simulink model "BMS_M0_pack_pass2"  (R2026a)
settings: Solver=VariableStepAuto  AbsTol=1e-3  EnableMultiTasking=on
undefined symbols (not defined in the file or in its folder): bat, mcu
libraries: fl_lib x22, nesl_utility x18, batteryecm_lib x6, ee_lib x4
settings SimscapeCC: SimscapeNominalValues="[{\"value\":\"1\",\"unit\":\"A\"},{\"value\":\"1\",\"unit\":\"bar\"},{\"value\":\"1\",\"unit\":\"cm^2\"},{\"value\":\"1\",\"unit\":\"cm^3/s\"},{\"value\":\"1\",\"unit\":\"kJ/kg\"},{\"value\":\"1\",\"unit\":\"kW\"},{\"value\":\"1\",\"unit\":\"l\"},{\"value\":\"1\",\"unit\":\"N\"},{\"value\":\"1\",\"unit\":\"N*m\"},{\"value\":\"1\",\"unit\":\"V\"}]"

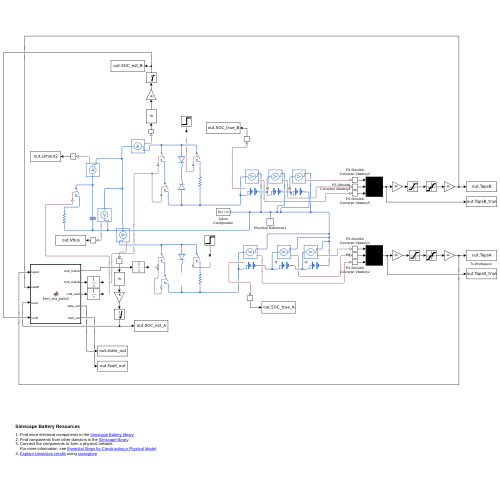
[thumbnail: Simulink's stored preview of the top-level diagram]
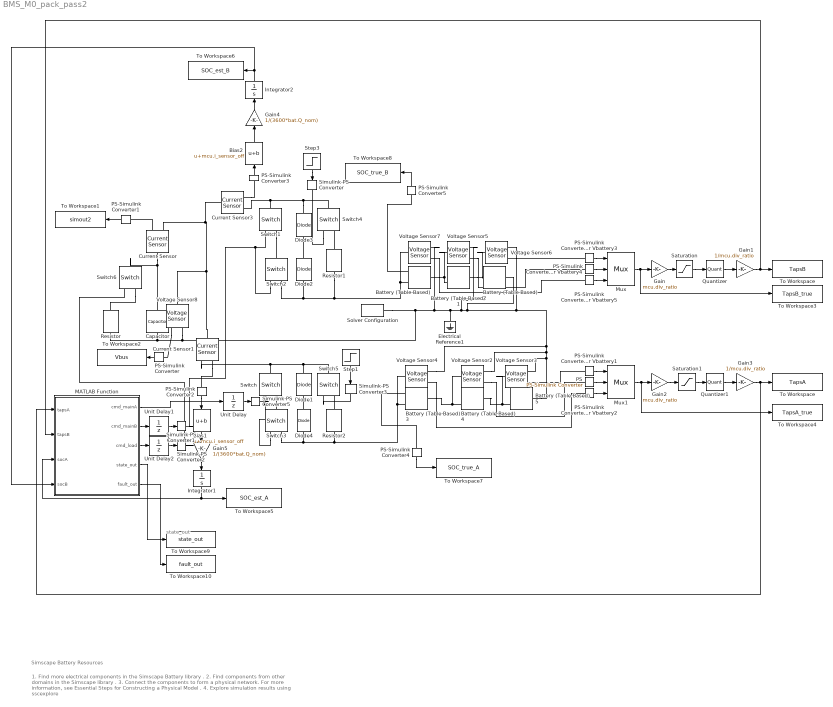
== system BMS_M0_pack_pass2 ==
  note: 1. Find more electrical components in the Simscape Battery library .
      | 2. Find components from other domains in the Simscape library .
      | 3. Connect the components to form a physical network.
      | For more information, see Essential Steps for Constructing a Physical Model .
      | 4. Explore simulation results using sscexplore
  note: Simscape Battery Resources
  note: state_out
  Battery (Table-Based){,1..3,5} (5 alike) : batteryecm_lib/Battery (Table-Based)  SOC_vec=bat.SOC_bp  T_dependence=simscape.enum.tablebattery.temperature_dependence.no  prm_dir=simscape.enum.tablebattery.prm_dir.noCurrentDirectionality  T_vec=[278, 293, 313] K  V0_mat=[3.49, 3.5, 3.51; 3.55, 3.57, 3.56; 3.62, 3.63, 3.64; 3.71, 3.71, 3.72; 3.91, 3.93, 3.94; 4.07, 4.08, 4.08; 4.19, 4.19, 4.19] V  V0_vec=bat.OCV_tbl V  V_range=[0, inf] V  R0_mat=[.0117, .0085, .009; .011, .0085, .009; .0114, .0087, .0092; .0107, .0082, .0088; .0107, .0083, .0091; .0113, .0085, .0089; .0116, .0085, .0089] Ohm  R0_vec=bat.R0 * ones(size(bat.SOC_bp)) Ohm  R0_dis_mat=[.0117, .0085, .009; .011, .0085, .009; .0114, .0087, .0092; .0107, .0082, .0088; .0107, .0083, .0091; .0113, .0085, .0089; .0116, .0085, .0089] Ohm  R0_dis_vec=[.0085, .0085, .0087, .0082, .0083, .0085, .0085] Ohm  R0_ch_mat=[.0117, .0085, .009; .011, .0085, .009; .0114, .0087, .0092; .0107, .0082, .0088; .0107, .0083, .0091; .0113, .0085, .0089; .0116, .0085, .0089] Ohm  R0_ch_vec=[.0085, .0085, .0087, .0082, .0083, .0085, .0085] Ohm  AH=bat.Q_nom A*hr  prm_leak=simscape.enum.tablebattery.prm_leak.disabled  Rleak_vec=[8000, 7000, 6000] Ohm  Rleak=7e3 Ohm  extrapolation_option=simscape.enum.extrapolation.nearest  SOC_port=simscape.enum.tablebattery.enable.yes  prm_dyn=simscape.enum.tablebattery.prm_dyn.off  R1_mat=[.0109, .0029, .0013; .0069, .0024, .0012; .0047, .0026, .0013; .0034, .0016, .001; .0033, .0023, .0014; .0033, .0018, .0011; .0028, .0017, .0011] Ohm  R1_vec=[.0029, .0024, .0026, .0016, .0023, .0018, .0017] Ohm  tau1_mat=[20, 36, 39; 31, 45, 39; 109, 105, 61; 36, 29, 26; 59, 77, 67; 40, 33, 29; 25, 39, 33] s  tau1_vec=[36, 45, 105, 29, 77, 33, 39] s  R2_mat=[.0109, .0029, .0013; .0069, .0024, .0012; .0047, .0026, .0013; .0034, .0016, .001; .0033, .0023, .0014; .0033, .0018, .0011; .0028, .0017, .0011] Ohm  R2_vec=[.0029, .0024, .0026, .0016, .0023, .0018, .0017] Ohm  tau2_mat=[20, 36, 39; 31, 45, 39; 109, 105, 61; 36, 29, 26; 59, 77, 67; 40, 33, 29; 25, 39, 33] s  tau2_vec=[36, 45, 105, 29, 77, 33, 39] s  R3_mat=[.0109, .0029, .0013; .0069, .0024, .0012; .0047, .0026, .0013; .0034, .0016, .001; .0033, .0023, .0014; .0033, .0018, .0011; .0028, .0017, .0011] Ohm  R3_vec=[.0029, .0024, .0026, .0016, .0023, .0018, .0017] Ohm  tau3_mat=[20, 36, 39; 31, 45, 39; 109, 105, 61; 36, 29, 26; 59, 77, 67; 40, 33, 29; 25, 39, 33] s  tau3_vec=[36, 45, 105, 29, 77, 33, 39] s  R4_mat=[.0109, .0029, .0013; .0069, .0024, .0012; .0047, .0026, .0013; .0034, .0016, .001; .0033, .0023, .0014; .0033, .0018, .0011; .0028, .0017, .0011] Ohm  R4_vec=[.0029, .0024, .0026, .0016, .0023, .0018, .0017] Ohm  tau4_mat=[20, 36, 39; 31, 45, 39; 109, 105, 61; 36, 29, 26; 59, 77, 67; 40, 33, 29; 25, 39, 33] s  tau4_vec=[36, 45, 105, 29, 77, 33, 39] s  R5_mat=[.0109, .0029, .0013; .0069, .0024, .0012; .0047, .0026, .0013; .0034, .0016, .001; .0033, .0023, .0014; .0033, .0018, .0011; .0028, .0017, .0011] Ohm  R5_vec=[.0029, .0024, .0026, .0016, .0023, .0018, .0017] Ohm  tau5_mat=[20, 36, 39; 31, 45, 39; 109, 105, 61; 36, 29, 26; 59, 77, 67; 40, 33, 29; 25, 39, 33] s  tau5_vec=[36, 45, 105, 29, 77, 33, 39] s  prm_fade=simscape.enum.tablebattery.prm_fade.disabled  N0=100  dV0=0  dR0=0  dAH=0  dRleak=0  dR1=0  dR2=0  dR3=0  dR4=0  dR5=0  N0vec=[0, 100, 200, 300]  Tfadevec=[298.15, 323.15] K  dV0vec=[0, 0, 0, 0]  dR0vec=[0, 0, 0, 0]  dAHvec=[0, 0, 0, 0]  dRleakvec=[0, 0, 0, 0]  dR1vec=[0, 0, 0, 0]  dR2vec=[0, 0, 0, 0]  dR3vec=[0, 0, 0, 0]  dR4vec=[0, 0, 0, 0]  dR5vec=[0, 0, 0, 0]  dV0mat=[0, 0; 0, 0; 0, 0; 0, 0]  dR0mat=[0, 0; 0, 0; 0, 0; 0, 0]  dAHmat=[0, 0; 0, 0; 0, 0; 0, 0]  dRleakmat=[0, 0; 0, 0; 0, 0; 0, 0]  dR1mat=[0, 0; 0, 0; 0, 0; 0, 0]  dR2mat=[0, 0; 0, 0; 0, 0; 0, 0]  dR3mat=[0, 0; 0, 0; 0, 0; 0, 0]  dR4mat=[0, 0; 0, 0; 0, 0; 0, 0]  dR5mat=[0, 0; 0, 0; 0, 0; 0, 0]  prm_age_modeling=simscape.enum.tablebattery.prm_age_modeling.equation  storage_dt_age_vec=[0] d  storage_T_age_vec=[273] K  prm_age_OCV=simscape.enum.tablebattery.prm_age_OCV.OCV  OCV_age=0.9  SOC_age=0.6  prm_age_resistance=simscape.enum.tablebattery.prm_age.disabled  OCV_scaling_age_resistance=2.2134e6  OCV_offset_age_resistance=1.632e6  temp_exp_age_resistance=0.515833569 V  t_exp_age_resistance=0.75  T_age_vec_resistance=[273.15, 298.15, 323.15] K  dt_age_vec_resistance=[0, 90, 180, 270] d  dR0_age_vec=[0, 0, 0]  t_meas_dR0_age=100 d  dR0_age_mat=[0, 0, 0; 0, 0, 0; 0, 0, 0; 0, 0, 0]  prm_age_capacity=simscape.enum.tablebattery.prm_age.disabled  OCV_scaling_age_capacity=1.5097e07  OCV_offset_age_capacity=8.3625e06  temp_exp_age_capacity=0.6011 V  t_exp_age_capacity=0.75  T_age_vec_capacity=[273.15, 298.15, 323.15] K  dt_age_vec_capacity=[0, 90, 180, 270] d  dAH_age_vec=[0, 0, 0]  t_meas_dAH_age=100 d  dAH_age_mat=[0, 0, 0; 0, 0, 0; 0, 0, 0; 0, 0, 0]  thermal_port=simscape.enum.thermaleffects.omit  temperature=298.15 K  thermal_mass=100 J/K  i_specify=off  i_priority=None  i=0 A  i_nominal_specify=off  i_nominal_value=1  i_nominal_unit=A  v_specify=off  v_priority=None  v=0 V  v_nominal_specify=off  v_nominal_value=1  v_nominal_unit=V  stateOfCharge_specify=on  stateOfCharge_priority=High  stateOfCharge=0.50  stateOfCharge_nominal_specify=off  stateOfCharge_nominal_value=1  stateOfCharge_nominal_unit=1  num_cycles_specify=off  num_cycles_priority=High  num_cycles=0  num_cycles_nominal_specify=off  num_cycles_nominal_value=1  num_cycles_nominal_unit=1  cell_temperature_specify=off  cell_temperature_priority=High  cell_temperature=298.15 K  cell_temperature_nominal_specify=off  cell_temperature_nominal_value=1  cell_temperature_nominal_unit=K
      settings: LibrarySourceBlock=|
      | batt_lib/Cells/Battery
      | (Table-Based)
  Battery (Table-Based)4 : batteryecm_lib/Battery (Table-Based)  SOC_vec=bat.SOC_bp  T_dependence=simscape.enum.tablebattery.temperature_dependence.no  prm_dir=simscape.enum.tablebattery.prm_dir.noCurrentDirectionality  T_vec=[278, 293, 313] K  V0_mat=[3.49, 3.5, 3.51; 3.55, 3.57, 3.56; 3.62, 3.63, 3.64; 3.71, 3.71, 3.72; 3.91, 3.93, 3.94; 4.07, 4.08, 4.08; 4.19, 4.19, 4.19] V  V0_vec=bat.OCV_tbl V  V_range=[0, inf] V  R0_mat=[.0117, .0085, .009; .011, .0085, .009; .0114, .0087, .0092; .0107, .0082, .0088; .0107, .0083, .0091; .0113, .0085, .0089; .0116, .0085, .0089] Ohm  R0_vec=bat.R0 * ones(size(bat.SOC_bp)) Ohm  R0_dis_mat=[.0117, .0085, .009; .011, .0085, .009; .0114, .0087, .0092; .0107, .0082, .0088; .0107, .0083, .0091; .0113, .0085, .0089; .0116, .0085, .0089] Ohm  R0_dis_vec=[.0085, .0085, .0087, .0082, .0083, .0085, .0085] Ohm  R0_ch_mat=[.0117, .0085, .009; .011, .0085, .009; .0114, .0087, .0092; .0107, .0082, .0088; .0107, .0083, .0091; .0113, .0085, .0089; .0116, .0085, .0089] Ohm  R0_ch_vec=[.0085, .0085, .0087, .0082, .0083, .0085, .0085] Ohm  AH=bat.Q_nom A*hr  prm_leak=simscape.enum.tablebattery.prm_leak.disabled  Rleak_vec=[8000, 7000, 6000] Ohm  Rleak=7e3 Ohm  extrapolation_option=simscape.enum.extrapolation.nearest  SOC_port=simscape.enum.tablebattery.enable.yes  prm_dyn=simscape.enum.tablebattery.prm_dyn.off  R1_mat=[.0109, .0029, .0013; .0069, .0024, .0012; .0047, .0026, .0013; .0034, .0016, .001; .0033, .0023, .0014; .0033, .0018, .0011; .0028, .0017, .0011] Ohm  R1_vec=[.0029, .0024, .0026, .0016, .0023, .0018, .0017] Ohm  tau1_mat=[20, 36, 39; 31, 45, 39; 109, 105, 61; 36, 29, 26; 59, 77, 67; 40, 33, 29; 25, 39, 33] s  tau1_vec=[36, 45, 105, 29, 77, 33, 39] s  R2_mat=[.0109, .0029, .0013; .0069, .0024, .0012; .0047, .0026, .0013; .0034, .0016, .001; .0033, .0023, .0014; .0033, .0018, .0011; .0028, .0017, .0011] Ohm  R2_vec=[.0029, .0024, .0026, .0016, .0023, .0018, .0017] Ohm  tau2_mat=[20, 36, 39; 31, 45, 39; 109, 105, 61; 36, 29, 26; 59, 77, 67; 40, 33, 29; 25, 39, 33] s  tau2_vec=[36, 45, 105, 29, 77, 33, 39] s  R3_mat=[.0109, .0029, .0013; .0069, .0024, .0012; .0047, .0026, .0013; .0034, .0016, .001; .0033, .0023, .0014; .0033, .0018, .0011; .0028, .0017, .0011] Ohm  R3_vec=[.0029, .0024, .0026, .0016, .0023, .0018, .0017] Ohm  tau3_mat=[20, 36, 39; 31, 45, 39; 109, 105, 61; 36, 29, 26; 59, 77, 67; 40, 33, 29; 25, 39, 33] s  tau3_vec=[36, 45, 105, 29, 77, 33, 39] s  R4_mat=[.0109, .0029, .0013; .0069, .0024, .0012; .0047, .0026, .0013; .0034, .0016, .001; .0033, .0023, .0014; .0033, .0018, .0011; .0028, .0017, .0011] Ohm  R4_vec=[.0029, .0024, .0026, .0016, .0023, .0018, .0017] Ohm  tau4_mat=[20, 36, 39; 31, 45, 39; 109, 105, 61; 36, 29, 26; 59, 77, 67; 40, 33, 29; 25, 39, 33] s  tau4_vec=[36, 45, 105, 29, 77, 33, 39] s  R5_mat=[.0109, .0029, .0013; .0069, .0024, .0012; .0047, .0026, .0013; .0034, .0016, .001; .0033, .0023, .0014; .0033, .0018, .0011; .0028, .0017, .0011] Ohm  R5_vec=[.0029, .0024, .0026, .0016, .0023, .0018, .0017] Ohm  tau5_mat=[20, 36, 39; 31, 45, 39; 109, 105, 61; 36, 29, 26; 59, 77, 67; 40, 33, 29; 25, 39, 33] s  tau5_vec=[36, 45, 105, 29, 77, 33, 39] s  prm_fade=simscape.enum.tablebattery.prm_fade.disabled  N0=100  dV0=0  dR0=0  dAH=0  dRleak=0  dR1=0  dR2=0  dR3=0  dR4=0  dR5=0  N0vec=[0, 100, 200, 300]  Tfadevec=[298.15, 323.15] K  dV0vec=[0, 0, 0, 0]  dR0vec=[0, 0, 0, 0]  dAHvec=[0, 0, 0, 0]  dRleakvec=[0, 0, 0, 0]  dR1vec=[0, 0, 0, 0]  dR2vec=[0, 0, 0, 0]  dR3vec=[0, 0, 0, 0]  dR4vec=[0, 0, 0, 0]  dR5vec=[0, 0, 0, 0]  dV0mat=[0, 0; 0, 0; 0, 0; 0, 0]  dR0mat=[0, 0; 0, 0; 0, 0; 0, 0]  dAHmat=[0, 0; 0, 0; 0, 0; 0, 0]  dRleakmat=[0, 0; 0, 0; 0, 0; 0, 0]  dR1mat=[0, 0; 0, 0; 0, 0; 0, 0]  dR2mat=[0, 0; 0, 0; 0, 0; 0, 0]  dR3mat=[0, 0; 0, 0; 0, 0; 0, 0]  dR4mat=[0, 0; 0, 0; 0, 0; 0, 0]  dR5mat=[0, 0; 0, 0; 0, 0; 0, 0]  prm_age_modeling=simscape.enum.tablebattery.prm_age_modeling.equation  storage_dt_age_vec=[0] d  storage_T_age_vec=[273] K  prm_age_OCV=simscape.enum.tablebattery.prm_age_OCV.OCV  OCV_age=0.9  SOC_age=0.6  prm_age_resistance=simscape.enum.tablebattery.prm_age.disabled  OCV_scaling_age_resistance=2.2134e6  OCV_offset_age_resistance=1.632e6  temp_exp_age_resistance=0.515833569 V  t_exp_age_resistance=0.75  T_age_vec_resistance=[273.15, 298.15, 323.15] K  dt_age_vec_resistance=[0, 90, 180, 270] d  dR0_age_vec=[0, 0, 0]  t_meas_dR0_age=100 d  dR0_age_mat=[0, 0, 0; 0, 0, 0; 0, 0, 0; 0, 0, 0]  prm_age_capacity=simscape.enum.tablebattery.prm_age.disabled  OCV_scaling_age_capacity=1.5097e07  OCV_offset_age_capacity=8.3625e06  temp_exp_age_capacity=0.6011 V  t_exp_age_capacity=0.75  T_age_vec_capacity=[273.15, 298.15, 323.15] K  dt_age_vec_capacity=[0, 90, 180, 270] d  dAH_age_vec=[0, 0, 0]  t_meas_dAH_age=100 d  dAH_age_mat=[0, 0, 0; 0, 0, 0; 0, 0, 0; 0, 0, 0]  thermal_port=simscape.enum.thermaleffects.omit  temperature=298.15 K  thermal_mass=100 J/K  i_specify=off  i_priority=None  i=0 A  i_nominal_specify=off  i_nominal_value=1  i_nominal_unit=A  v_specify=off  v_priority=None  v=0 V  v_nominal_specify=off  v_nominal_value=1  v_nominal_unit=V  stateOfCharge_specify=on  stateOfCharge_priority=High  stateOfCharge=0.20  stateOfCharge_nominal_specify=off  stateOfCharge_nominal_value=1  stateOfCharge_nominal_unit=1  num_cycles_specify=off  num_cycles_priority=High  num_cycles=0  num_cycles_nominal_specify=off  num_cycles_nominal_value=1  num_cycles_nominal_unit=1  cell_temperature_specify=off  cell_temperature_priority=High  cell_temperature=298.15 K  cell_temperature_nominal_specify=off  cell_temperature_nominal_value=1  cell_temperature_nominal_unit=K
      settings: LibrarySourceBlock=|
      | batt_lib/Cells/Battery
      | (Table-Based)
  Bias1 : Bias  Bias=mcu.i_sensor_off  SaturateOnIntegerOverflow=off
  Bias2 : Bias  Bias=mcu.i_sensor_off  SaturateOnIntegerOverflow=off
  Capacitor : fl_lib/Electrical/Electrical Elements/Capacitor  c=1000 uF  r=1e-6 Ohm  g=0 1/Ohm  i_specify=off  i_priority=None  i=0 A  i_nominal_specify=off  i_nominal_value=1  i_nominal_unit=A  v_specify=off  v_priority=None  v=0 V  v_nominal_specify=off  v_nominal_value=1  v_nominal_unit=V  vc_specify=off  vc_priority=High  vc=0 V  vc_nominal_specify=off  vc_nominal_value=1  vc_nominal_unit=V
  Current Sensor : fl_lib/Electrical/Electrical Sensors/Current Sensor
  Current Sensor1 : fl_lib/Electrical/Electrical Sensors/Current Sensor
  Current Sensor3 : fl_lib/Electrical/Electrical Sensors/Current Sensor
  Diode{1..4} (4 alike) : ee_lib/Semiconductors & Converters/Diode  ModelType=ee.enum.diode.modelType.pwl  TableType=ee.enum.diode.tableType.IfMat  IfMat=[.07, .12, .19, 1.75, 4.24, 7.32, 11.2; .16, .3, .72, 2.14, 5.02, 8.35, 13.12] A  VfMat=[.9, 1.15, 1.25, 1.5, 1.75, 2.17, 2.6, 2.85; .58, .68, .75, 1.1, 1.38, 1.77, 2.27, 2.7] V  TjVec=[25, 125] degC  VfVec=[.5, .7, .9, 1.3, 1.7, 2.1, 2.5] V  IfVec=[.1, .2, .5, 1, 2, 4, 7, 10] A  IrMat=[1e-06, 2e-06, 5e-06, 1e-05, 2.5e-05, 5e-05, .0001; 2e-06, 5e-06, 1e-05, 4e-05, 8e-05, .0002, .0005] A  VrMat=[10, 100, 200, 250, 300, 325, 350; 10, 70, 160, 220, 270, 300, 320] V  VrVec=[10, 20, 40, 50, 70, 80, 100] V  IrVec=[1e-06, 2e-06, 5e-06, 1e-05, 2e-05, 5e-05, .0001] A  Vf=0.8 V  Ron=0.01 Ohm  Goff=1e-8 S  prmExp=ee.enum.diode.expParam.useTwo  I12=[.0137, .545] A  V12=[.6, .7] V  RS=0 Ohm  Tmeas=298.15 K  IS=1e-12 A  ec=1  I1=0.0137 A  V1=0.6 V  N_series=1  N_parallel=1  ZenerEnable=false  Rz=0.3 Ohm  BV=30 V  C_param=ee.enum.diode.capParam.fixed  CJ=0 pF  CJ0=5 pF  Vvec=[.1, 10, 100] V  Cvec=[3.5, 1, .4] pF  VJ=1 V  Mgrad=0.5  FC=0.5  Q_param=ee.enum.diode.recoveryParam.off  iRM=-7.15 A  iF=4 A  didt=-750 A/us  trr_factor=3  trr=115 ns  Qrr=150 nA*s  Vr=-600 V  Ls=150 nH  Erec=0.03 J  TT=50 ns  tau=100 ns  T_param=ee.enum.diode.temperatureParam.off  Tdevice=298.15 K  I1_T2=0.245 A  V1_T2=0.5 V  IS_T2=1.25e-7 A  Tmeas2=125 degC  XTI_param=ee.enum.diode.xtiParam.pn  XTI=3  EG_param=ee.enum.diode.egapParam.material_si  EG=1.11 eV  dBVdT=0 V/K  enable_fault_input=simscape.enum.onoff.off  i_specify=off  i_priority=None  i=0 A  i_nominal_specify=off  i_nominal_value=1  i_nominal_unit=A  v_specify=off  v_priority=None  v=0 V  v_nominal_specify=off  v_nominal_value=1  v_nominal_unit=V  v_capacitor_specify=off  v_capacitor_priority=None  v_capacitor=0 V  v_capacitor_nominal_specify=off  v_capacitor_nominal_value=1  v_capacitor_nominal_unit=V  Qj_specify=off  Qj_priority=High  Qj=0 C  Qj_nominal_specify=off  Qj_nominal_value=1  Qj_nominal_unit=C  i_diode_specify=off  i_diode_priority=None  i_diode=0 A  i_diode_nominal_specify=off  i_diode_nominal_value=1  i_diode_nominal_unit=A  v_diode_specify=off  v_diode_priority=None  v_diode=0 V  v_diode_nominal_specify=off  v_diode_nominal_value=1  v_diode_nominal_unit=V  i_capacitor_specify=off  i_capacitor_priority=None  i_capacitor=0 A  i_capacitor_nominal_specify=off  i_capacitor_nominal_value=1  i_capacitor_nominal_unit=A  fidelity_level=ee.enum.diode.fidelity.includeChargeDyn  rec_loss_model=ee.enum.diode.reverseRecoveryModelTabulateUpTo3D.fixed  ErecVal=0 J  scaleWithIandV=true  ErecMat=zeros(2, 3) J  ErecMat3D=zeros(2, 3, 2) J  TjrecVec=[298.15, 398.15] K  IfrecVec=[.1, 1, 10] A  IrecVal=10 A  VrecVal=10 V  VrecVec=[0, 100] V  tFilter=1 / 1000 / 100 s  thermal_network_parameterization=ee.enum.thermalNetworkTopology.junctionCase  Rth=[0, 10] K/W  Rth_Cauer=[1, 3, 10] K/W  Rth_Foster=[.08, .14, .22, .16] K/W  thermal_mass_parameterization=ee.enum.thermalNetwork.timeconstant  thermal_mass=[0, 1] J/K  thermal_mass_Cauer=[.1, .3, 1] J/K  thermal_mass_Foster=[.001, .005, .05, .5] J/K  thermal_time_constant=[0, 10] s  thermal_time_constant_Cauer=[1, 3, 10] s  thermal_time_constant_Foster=[7e-05, .0007, .01, .08] s  thermal_mass_initial_temperatures=[25, 25] degC  thermal_mass_initial_temperatures_Cauer=[25, 25, 25] degC  junction_thermal_mass=0.01 J/K  Tvec_initial_Foster=[25, 25, 25, 25] degC  no_thermal_network=0  junction_temperature_specify=off  junction_temperature_priority=None  junction_temperature=25 degC  junction_temperature_nominal_specify=off  junction_temperature_nominal_value=1  junction_temperature_nominal_unit=degC
  Electrical Reference1 : fl_lib/Electrical/Electrical Elements/Electrical Reference
  Gain : Gain  Gain=mcu.div_ratio
  Gain1 : Gain  Gain=1/mcu.div_ratio
  Gain2 : Gain  Gain=mcu.div_ratio
  Gain3 : Gain  Gain=1/mcu.div_ratio
  Gain4 : Gain  Gain=1/(3600*bat.Q_nom)
  Gain5 : Gain  Gain=1/(3600*bat.Q_nom)
  Integrator1 : Integrator  InitialCondition=0.55  LimitOutput=on  UpperSaturationLimit=1  LowerSaturationLimit=0
  Integrator2 : Integrator  InitialCondition=0.55  LimitOutput=on  UpperSaturationLimit=1  LowerSaturationLimit=0
  MATLAB Function : MATLAB Function  TreatAsAtomicUnit=on  SystemSampleTime=0.1
  Mux : Mux  Inputs=3
  Mux1 : Mux  Inputs=3
  PS : nesl_utility/PS-Simulink Converter  PhysicalDomain=network_engine_domain  SubClassName=ps_output  LeftPortType=input  RightPortType=output  PseudoPeriodic=off  Frequencies=[]  VectorFormat=inherit  Unit=inherit  AffineConversion=off
  PS-Simulink Converter{,1..5} (6 alike) : nesl_utility/PS-Simulink Converter  PhysicalDomain=network_engine_domain  SubClassName=ps_output  LeftPortType=input  RightPortType=output  PseudoPeriodic=off  Frequencies=[]  VectorFormat=inherit  Unit=inherit  AffineConversion=off
  PS-Simulink Converter Vbattery{1..5} (5 alike) : nesl_utility/PS-Simulink Converter  PhysicalDomain=network_engine_domain  SubClassName=ps_output  LeftPortType=input  RightPortType=output  PseudoPeriodic=off  Frequencies=[]  VectorFormat=inherit  Unit=inherit  AffineConversion=off
  Quantizer : Quantizer  QuantizationInterval=mcu.lsb_adc
  Quantizer1 : Quantizer  QuantizationInterval=mcu.lsb_adc
  Resistor : fl_lib/Electrical/Electrical Elements/Resistor  R=2.2 Ohm  i_specify=off  i_priority=None  i=0 A  i_nominal_specify=off  i_nominal_value=1  i_nominal_unit=A  v_specify=off  v_priority=None  v=0 V  v_nominal_specify=off  v_nominal_value=1  v_nominal_unit=V
  Resistor1 : fl_lib/Electrical/Electrical Elements/Resistor  R=10 Ohm  i_specify=off  i_priority=None  i=0 A  i_nominal_specify=off  i_nominal_value=1  i_nominal_unit=A  v_specify=off  v_priority=None  v=0 V  v_nominal_specify=off  v_nominal_value=1  v_nominal_unit=V
  Resistor2 : fl_lib/Electrical/Electrical Elements/Resistor  R=10 Ohm  i_specify=off  i_priority=None  i=0 A  i_nominal_specify=off  i_nominal_value=1  i_nominal_unit=A  v_specify=off  v_priority=None  v=0 V  v_nominal_specify=off  v_nominal_value=1  v_nominal_unit=V
  Saturation : Saturate  UpperLimit=3.3  LowerLimit=0
  Saturation1 : Saturate  UpperLimit=3.3  LowerLimit=0
  Simulink-PS Converter{,1..3,5} (5 alike) : nesl_utility/Simulink-PS Converter  PhysicalDomain=network_engine_domain  SubClassName=ps_input  LeftPortType=input  RightPortType=output  PseudoPeriodic=off  Frequencies=[]  NoiseDistribution=none  NoiseParameters=[]  Unit=1  AffineConversion=off  FilteringAndDerivatives=provide  SimscapeFilterOrder=1  InputFilterTimeConstant=0.001  UdotUserProvided=0
  Solver Configuration : nesl_utility/Solver Configuration  PhysicalDomain=network_engine_domain  SubClassName=solver  LeftPortType=input  RightPortType=generic  Tones=[]  Harmonics=[]  SimulateNoise=off  Profile=off  UseLocalSampling=off  EnableSwitchedLinearOptims=on  FrequencyDomain=off  UseCCode=off  RelTol=0.001  AbsTol=1e-06  MinStep=1e-09  ToWorkspace=off  RevertToSquareIcSolve=off  NumHomotopyIterations=100  PhasorMode=off  PhasorModeNumHarmonics=1  ConsistencySolver=NEWTON_XTOL_AFTER_FTOL  CanonicalOrdering=UNORDERED  OptimizeIntermediates=UNOPTIMIZED  IndexReductionMethod=DerivativeReplacement  DoDC=off  ResidualTolerance=1e-09  ConsistencyTolSource=GLOBAL  ConsistencyAbsTol=0.001  ConsistencyRelTol=0.001  ConsistencyTolFactor=0.001  UseLocalSolver=off  LocalSolverChoice=NE_BACKWARD_EULER_ADVANCER  ResolveIndetEquations=on  FunctionEvalNumThread=1  LocalSolverSampleTime=0.001  DoFixedCost=off  MaxNonlinIter=3  MaxModeIter=2  ComputeImpulses=off  ImpulseIterations=2  LinearAlgebra=auto  LinearAlgebraNumThread=0  EquationFormulation=NE_TIME_EF  DelaysMemoryBudget=1024  AutomaticFiltering=on  FilteringTimeConstant=0.001  PartitionStorageMethod=AS_NEEDED  PartitionMemoryBudget=1024  PartitionMethod=ROBUST  MultibodyUseLocalSolver=off  MultibodyLocalSolverChoice=ODE1  MultibodyLocalSolverSampleTime=0.001
  Step1 : Step  Time=0.001  SampleTime=0
  Step3 : Step  Time=0.001  FinalValue=0  SampleTime=0
  Switch{,1..3,6} (5 alike) : fl_lib/Electrical/Electrical Elements/Switch  R_closed=fet.Rds_on Ohm  G_open=1e-8 1/Ohm  Threshold=0.5  i_specify=off  i_priority=None  i=0 A  i_nominal_specify=off  i_nominal_value=1  i_nominal_unit=A  v_specify=off  v_priority=None  v=0 V  v_nominal_specify=off  v_nominal_value=1  v_nominal_unit=V
  Switch4 : fl_lib/Electrical/Electrical Elements/Switch  R_closed=0.01 Ohm  G_open=1e-8 1/Ohm  Threshold=0.5  i_specify=off  i_priority=None  i=0 A  i_nominal_specify=off  i_nominal_value=1  i_nominal_unit=A  v_specify=off  v_priority=None  v=0 V  v_nominal_specify=off  v_nominal_value=1  v_nominal_unit=V
  Switch5 : fl_lib/Electrical/Electrical Elements/Switch  R_closed=0.01 Ohm  G_open=1e-8 1/Ohm  Threshold=0.5  i_specify=off  i_priority=None  i=0 A  i_nominal_specify=off  i_nominal_value=1  i_nominal_unit=A  v_specify=off  v_priority=None  v=0 V  v_nominal_specify=off  v_nominal_value=1  v_nominal_unit=V
  To Workspace : ToWorkspace  VariableName=TapsB  SaveFormat=Timeseries  SampleTime=-1
  "To Workspace " : ToWorkspace  VariableName=TapsA  SaveFormat=Timeseries  SampleTime=-1
  To Workspace1 : ToWorkspace  VariableName=simout2  SaveFormat=Timeseries  SampleTime=-1
  To Workspace10 : ToWorkspace  VariableName=fault_out  SaveFormat=Timeseries  SampleTime=-1
  To Workspace2 : ToWorkspace  VariableName=Vbus  SaveFormat=Timeseries  SampleTime=-1
  To Workspace3 : ToWorkspace  VariableName=TapsB_true  SaveFormat=Timeseries  SampleTime=-1
  To Workspace4 : ToWorkspace  VariableName=TapsA_true  SaveFormat=Timeseries  SampleTime=-1
  To Workspace5 : ToWorkspace  VariableName=SOC_est_A  SaveFormat=Timeseries  SampleTime=-1
  To Workspace6 : ToWorkspace  VariableName=SOC_est_B  SaveFormat=Timeseries  SampleTime=-1
  To Workspace7 : ToWorkspace  VariableName=SOC_true_A  SaveFormat=Timeseries  SampleTime=-1
  To Workspace8 : ToWorkspace  VariableName=SOC_true_B  SaveFormat=Timeseries  SampleTime=-1
  To Workspace9 : ToWorkspace  VariableName=state_out  SaveFormat=Timeseries  SampleTime=-1
  Unit Delay : UnitDelay  SampleTime=0.1
  Unit Delay1 : UnitDelay  SampleTime=0.1
  Unit Delay2 : UnitDelay  SampleTime=0.1
  Voltage Sensor{2..8} (7 alike) : fl_lib/Electrical/Electrical Sensors/Voltage Sensor
  wires:
  PS-Simulink Converter Vbattery1/1 -> Mux1/1
  Gain4/1 -> Integrator2/1
  Unit Delay1/1 -> Simulink-PS Converter1/1
  Step3/1 -> Simulink-PS Converter/1
  Gain2/1 -> Saturation1/1
  Bias2/1 -> Gain4/1
  Saturation1/1 -> Quantizer1/1
  PS-Simulink Converter/1 -> To Workspace2/1
  PS-Simulink Converter Vbattery2/1 -> Mux1/3
  PS-Simulink Converter Vbattery5/1 -> Mux/3
  Gain5/1 -> Integrator1/1
  PS-Simulink Converter Vbattery4/1 -> Mux/2
  Gain1/1 -> MATLAB Function/2(tapsB), To Workspace/1
  Integrator2/1 -> MATLAB Function/4(socB), To Workspace6/1
  Unit Delay2/1 -> Simulink-PS Converter2/1
  MATLAB Function/4(state_out) -> To Workspace9/1
  Integrator1/1 -> To Workspace5/1, MATLAB Function/3(socA)
  MATLAB Function/2(cmd_mainB) -> Unit Delay1/1
  PS-Simulink Converter4/1 -> To Workspace7/1
  Saturation/1 -> Quantizer/1
  PS-Simulink Converter1/1 -> To Workspace1/1
  MATLAB Function/3(cmd_load) -> Unit Delay2/1
  MATLAB Function/5(fault_out) -> To Workspace10/1
  Gain/1 -> Saturation/1
  PS-Simulink Converter Vbattery3/1 -> Mux/1
  PS-Simulink Converter2/1 -> Bias1/1
  Mux/1 -> To Workspace3/1, Gain/1
  Quantizer/1 -> Gain1/1
  Unit Delay/1 -> Simulink-PS Converter5/1
  Quantizer1/1 -> Gain3/1
  PS-Simulink Converter5/1 -> To Workspace8/1
  Step1/1 -> Simulink-PS Converter3/1
  Gain3/1 -> MATLAB Function/1(tapsA), "To Workspace "/1
  PS/1 -> Mux1/2
  MATLAB Function/1(cmd_mainA) -> Unit Delay/1
  Bias1/1 -> Gain5/1
  Mux1/1 -> To Workspace4/1, Gain2/1
  PS-Simulink Converter3/1 -> Bias2/1
  connections:
  Battery (Table-Based)1/RConn1 -- Voltage Sensor6/LConn1 -- Battery (Table-Based)2/LConn1
  Diode2/LConn1 -- Switch2/RConn2 -- Voltage Sensor7/LConn1 -- Battery (Table-Based)/LConn1 -- Resistor1/RConn1
  Battery (Table-Based)5/LConn1 -- Battery (Table-Based)4/RConn1 -- Voltage Sensor3/LConn1
  Battery (Table-Based)4/LConn1 -- Battery (Table-Based)3/RConn1 -- Voltage Sensor2/LConn1
  Voltage Sensor4/RConn2 -- Solver Configuration/RConn1 -- Resistor/RConn1 -- Capacitor/RConn1 -- Voltage Sensor8/RConn2 -- Voltage Sensor7/RConn2 -- Electrical Reference1/LConn1 -- Voltage Sensor5/RConn2 -- Battery (Table-Based)2/RConn1 -- Voltage Sensor6/RConn2 -- Battery (Table-Based)5/RConn1 -- Voltage Sensor3/RConn2 -- Voltage Sensor2/RConn2
  Battery (Table-Based)3/LConn1 -- Resistor2/RConn1 -- Diode4/LConn1 -- Switch3/RConn2 -- Voltage Sensor4/LConn1
  Diode3/LConn1 -- Switch1/LConn1 -- Current Sensor3/RConn2 -- Switch4/LConn1
  Voltage Sensor8/LConn1 -- Current Sensor1/LConn1 -- Current Sensor/RConn2 -- Current Sensor3/LConn1
  Diode1/LConn1 -- Switch5/LConn1 -- Switch/LConn1 -- Current Sensor1/RConn2
  Battery (Table-Based)/RConn1 -- Battery (Table-Based)1/LConn1 -- Voltage Sensor5/LConn1
  Switch6/LConn1 -- Current Sensor/LConn1 -- Capacitor/LConn1
  Simulink-PS Converter1/RConn1 -- Switch2/RConn1 -- Switch1/RConn1
  Switch/RConn1 -- Simulink-PS Converter5/RConn1 -- Switch3/RConn1
  PS-Simulink Converter4/LConn1 -- Battery (Table-Based)3/LConn2
  Diode4/RConn1 -- Diode1/RConn1
  Switch6/RConn2 -- Resistor/LConn1
  Voltage Sensor2/RConn1 -- PS/LConn1
  Voltage Sensor5/RConn1 -- PS-Simulink Converter Vbattery4/LConn1
  Voltage Sensor8/RConn1 -- PS-Simulink Converter/LConn1
  Voltage Sensor6/RConn1 -- PS-Simulink Converter Vbattery3/LConn1
  Switch5/RConn1 -- Simulink-PS Converter3/RConn1
  Resistor2/LConn1 -- Switch5/RConn2
  Diode2/RConn1 -- Diode3/RConn1
  Simulink-PS Converter2/RConn1 -- Switch6/RConn1
  Current Sensor1/RConn1 -- PS-Simulink Converter2/LConn1
  Resistor1/LConn1 -- Switch4/RConn2
  Voltage Sensor3/RConn1 -- PS-Simulink Converter Vbattery1/LConn1
  Switch1/RConn2 -- Switch2/LConn1
  Switch4/RConn1 -- Simulink-PS Converter/RConn1
  Current Sensor3/RConn1 -- PS-Simulink Converter3/LConn1
  Switch/RConn2 -- Switch3/LConn1
  Voltage Sensor7/RConn1 -- PS-Simulink Converter Vbattery5/LConn1
  Voltage Sensor4/RConn1 -- PS-Simulink Converter Vbattery2/LConn1
  Battery (Table-Based)/LConn2 -- PS-Simulink Converter5/LConn1
  Current Sensor/RConn1 -- PS-Simulink Converter1/LConn1

== matlab function BMS_M0_pack_pass2/MATLAB Function ==
  data: tapsA input; cmd_mainA output; tapsB input; socA input; socB input; cmd_mainB output; cmd_load output; state_out output; fault_out output
function [cmd_mainA, cmd_mainB, cmd_load, state_out, fault_out] = ...
         bms_soa_pass2(tapsA, tapsB, socA, socB)
%BMS_SOA_PASS2  Safe-operating-area layer for reconfigurable 3S2P BMS.
%
%  MILESTONE 0 -- PASS 2.  Safety checks only. No topology optimisation,
%  no precharge sequencing, no cooldown. Those are Pass 3.
%
%  DESIGN RULE (from project brief): SOA checks run BEFORE any efficiency
%  or balancing logic. A string that violates SOA is isolated regardless
%  of what the SOC logic would prefer.
%
%  INPUTS
%    tapsA, tapsB  3x1  quantised tap voltages, referenced to pack negative.
%                       These are what the ADC actually returns after the
%                       33k/10k divider. Per-cell voltage is NOT measured
%                       directly -- it is reconstructed below by subtraction,
%                       exactly as the STM32 firmware will do it.
%    socA, socB    1x1  coulomb-counted SOC ESTIMATES. Never the simulator's
%                       true SOC -- the MCU cannot know that.
%
%  OUTPUTS
%    cmd_mainA/B   0/1  main switch pair command per string
%    cmd_load      0/1  load disconnect switch
%    state_out          see state codes below
%    fault_out          bitfield, see fault codes below
%
%  NOTE ON ISOLATED STRINGS: the tap dividers are permanently connected to
%  the cells, so an isolated string still reports valid (open-circuit) tap
%  voltages. This mirrors the hardware and means we can keep monitoring a
%  string we have disconnected.

%% ---- CONSTANTS -----------------------------------------------------
% KEEP IN SYNC WITH BMS_params.m. A MATLAB Function block cannot read the
% base workspace, so these are duplicated. If you change a threshold there,
% change it here too.
V_UV_TRIP   = 2.50;   % V  [VERIFIED] SPEC pack design guideline, NCA
V_OV_TRIP   = 4.20;   % V  [VERIFIED] SPEC 3.3, cell absolute max
V_UV_WARN   = 2.80;   % V  [ASSUMPTION] margin above trip
DEBOUNCE_N  = 3;      %    [ASSUMPTION] consecutive samples before tripping
                      %    3 samples at 100 ms = 300 ms. Long enough to
                      %    reject a single quantisation flicker, short
                      %    enough to act well before cell damage.

%% ---- STATE CODES ---------------------------------------------------
S_INIT      = 0;
S_BOTH      = 1;   % both strings carrying load
S_ISOLATE_A = 2;   % A faulted, B carries load
S_ISOLATE_B = 3;   % B faulted, A carries load
S_SHUTDOWN  = 4;   % both faulted -- LATCHED, no auto-recovery

%% ---- FAULT BITS ----------------------------------------------------
F_NONE   = 0;
F_UV_A   = 1;    % bit 0
F_UV_B   = 2;    % bit 1
F_OV_A   = 4;    % bit 2
F_OV_B   = 8;    % bit 3

%% ---- PERSISTENT STATE ----------------------------------------------
% These survive between 100 ms calls, exactly like static variables in C.
persistent state fault uvA_cnt uvB_cnt ovA_cnt ovB_cnt

if isempty(state)
    % POWER-UP DEFAULT: all switches OFF.
    % Mirrors the 100k base pull-downs on the 2N2222A gate drivers -- on
    % reset or brownout the hardware defaults to open, and so does this.
    state   = S_INIT;
    fault   = F_NONE;
    uvA_cnt = 0;  uvB_cnt = 0;
    ovA_cnt = 0;  ovB_cnt = 0;
end

%% ---- RECONSTRUCT PER-CELL VOLTAGES ---------------------------------
% The firmware does this same subtraction. Measured error is ~0.4 mV
% typical, bounded near 7 mV worst case (2 LSB at 3.46 mV/LSB).
vA = [ tapsA(1);
       tapsA(2) - tapsA(1);
       tapsA(3) - tapsA(2) ];

vB = [ tapsB(1);
       tapsB(2) - tapsB(1);
       tapsB(3) - tapsB(2) ];

%% ---- SOA CHECKS, WITH DEBOUNCE -------------------------------------
% Debounce matters because a single sample straddling a quantisation
% boundary can read one LSB low. Tripping on that would cause spurious
% isolation -- the "false triggers will ruin the demo" failure mode.

uvA_now = any(vA < V_UV_TRIP);
uvB_now = any(vB < V_UV_TRIP);
ovA_now = any(vA > V_OV_TRIP);
ovB_now = any(vB > V_OV_TRIP);

if uvA_now, uvA_cnt = uvA_cnt + 1; else, uvA_cnt = 0; end
if uvB_now, uvB_cnt = uvB_cnt + 1; else, uvB_cnt = 0; end
if ovA_now, ovA_cnt = ovA_cnt + 1; else, ovA_cnt = 0; end
if ovB_now, ovB_cnt = ovB_cnt + 1; else, ovB_cnt = 0; end

% Faults LATCH. Once a string has violated SOA we do not re-close it on
% the strength of a later good reading -- an unloaded cell recovers voltage
% and would look healthy again, causing oscillation.
if uvA_cnt >= DEBOUNCE_N, fault = bitor(fault, F_UV_A); end
if uvB_cnt >= DEBOUNCE_N, fault = bitor(fault, F_UV_B); end
if ovA_cnt >= DEBOUNCE_N, fault = bitor(fault, F_OV_A); end
if ovB_cnt >= DEBOUNCE_N, fault = bitor(fault, F_OV_B); end

faultA = bitand(fault, bitor(F_UV_A, F_OV_A)) ~= 0;
faultB = bitand(fault, bitor(F_UV_B, F_OV_B)) ~= 0;

%% ---- STATE TRANSITIONS ---------------------------------------------
% Safety-driven only in Pass 2. SOC and balancing logic is Pass 3.
switch state

    case S_INIT
        if      faultA && faultB, state = S_SHUTDOWN;
        elseif  faultA,           state = S_ISOLATE_A;
        elseif  faultB,           state = S_ISOLATE_B;
        else,                     state = S_BOTH;
        end

    case S_BOTH
        if      faultA && faultB, state = S_SHUTDOWN;
        elseif  faultA,           state = S_ISOLATE_A;
        elseif  faultB,           state = S_ISOLATE_B;
        end

    case S_ISOLATE_A
        if faultB, state = S_SHUTDOWN; end   % last healthy string gone

    case S_ISOLATE_B
        if faultA, state = S_SHUTDOWN; end

    case S_SHUTDOWN
        % TERMINAL. No path out. A latched safety trip requires operator
        % reset -- auto-recovery from an unknown fault is not defensible.

    otherwise
        state = S_SHUTDOWN;   % unreachable; fail safe if it ever happens
end

%% ---- OUTPUTS -------------------------------------------------------
switch state
    case S_INIT,       cmd_mainA = 0; cmd_mainB = 0; cmd_load = 0;
    case S_BOTH,       cmd_mainA = 1; cmd_mainB = 1; cmd_load = 1;
    case S_ISOLATE_A,  cmd_mainA = 0; cmd_mainB = 1; cmd_load = 1;
    case S_ISOLATE_B,  cmd_mainA = 1; cmd_mainB = 0; cmd_load = 1;
    case S_SHUTDOWN,   cmd_mainA = 0; cmd_mainB = 0; cmd_load = 0;
    otherwise,         cmd_mainA = 0; cmd_mainB = 0; cmd_load = 0;
end

state_out = state;
fault_out = fault;

% Suppress unused-input warnings. socA/socB arrive now so the interface is
% stable when Pass 3 adds balancing logic.
socA = socA; %#ok<NASGU,ASGSL>
socB = socB; %#ok<NASGU,ASGSL>

end

%% =====================================================================
%  FMEA -- PASS 2
%  =====================================================================
%
%  FAILURE                  DETECTION                  SAFE RESPONSE
%  -----------------------------------------------------------------
%  Cell undervoltage        vA/vB < 2.50 V, 3 samples  Isolate that string;
%                                                      shutdown if both
%
%  Cell overvoltage         vA/vB > 4.20 V, 3 samples  Isolate that string
%
%  Tap sensor open circuit  Reads ~0 V, trips UV       Isolate. Fails safe,
%                                                      though it cannot be
%                                                      distinguished from a
%                                                      genuinely flat cell.
%                                                      [GAP -- see below]
%
%  Tap sensor short to rail Reads high, trips OV       Isolate
%
%  Both strings faulted     faultA && faultB           SHUTDOWN, latched,
%                                                      load disconnected
%
%  MCU reset mid-mission    persistent vars cleared    Re-enters S_INIT with
%                                                      all switches off; the
%                                                      100k pull-downs hold
%                                                      the hardware open
%                                                      through the reset
%
%  Quantisation flicker     Debounce counter resets    No spurious trip
%
%  KNOWN GAPS (Pass 3+):
%    - No overcurrent check       -> needs string current inputs
%    - No overtemperature check   -> needs temperature inputs
%    - No state validation        -> commands are not read back and
%                                    confirmed against measured current.
%                                    A welded-closed MOSFET is currently
%                                    undetectable. REQUIRED before M1.
%    - No cooldown timer          -> topology could oscillate
%    - No dV check before paralleling -> Pass 3
